simulink model "EChacks1"  (R2018a)
settings: Solver=FixedStepAuto  StartTime=0.0  StopTime=inf  RelTol=1e-3  EnableMultiTasking=on
PreLoadFcn:
  | Ts = 0.01;
  | Ts_wifi = 0.1;
libraries: arduinosensorlib x2, simulink x1
settings Model: SimulationMode=external  ExtModeTrigDuration=2  Creator=bnewman  LastModifiedBy=niuniusongqiang
settings OptimizationCC: PassReuseOutputArgsThreshold=0  MaxStackSize=64
settings DebuggingCC: ParameterTunabilityLossMsg=error
settings HardwareCC: ProdBitPerPointer=32  ProdBitPerSizeT=32  ProdBitPerPtrDiffT=32  ProdLargestAtomicInteger=Long  ProdLargestAtomicFloat=Double  ProdWordSize=32  ProdHWDeviceType=ARM Compatible->ARM Cortex  UseEmbeddedCoderFeatures=off  UseSimulinkCoderFeatures=off
settings SFSimCC: MATLABDynamicMemAlloc=off
settings RTWCC: SystemTargetFile=ert.tlc  HardwareBoard=Arduino MKR1000  TLCOptions=-aInlineSetEventsForThisBaseRateFcn=TLC_FALSE -aSuppressMultiTaskScheduler=TLC_FALSE -aRateBasedStepFcn=1  TemplateMakefile=ert_default_tmf  GenerateReport=on  Toolchain=Arduino ARM  BuildConfiguration=Faster Runs  LaunchReport=on
settings CodeAppCC: ForceParamTrailComments=on  OperatorAnnotations=on
settings ERTTargetCC: ERTCustomFileBanners=off  SupportContinuousTime=on  SupportNonInlinedSFcns=on  RemoveResetFunc=off  SupportVariableSizeSignals=on  ModelStepFunctionPrototypeControlCompliant=off

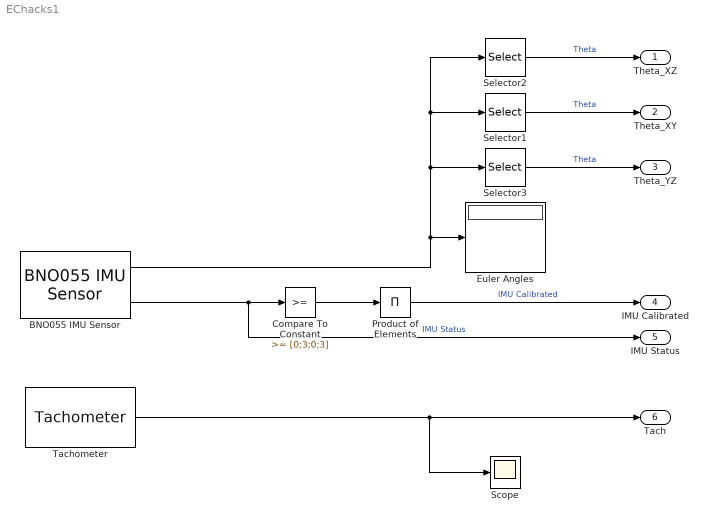
== system EChacks1 ==
  BNO055 IMU Sensor : arduinosensorlib/BNO055 IMU Sensor  SlaveAddress=0x28  OperationMode=Fusion  SlaveAddress_=hex2dec( '28' )  Accel=off  AngularRate=off  MagField=off  EulerAngles=on  Quat=off  LinearAccel=off  GravityVector=off  AccelRange=4G  AccelBW=62.5 Hz  GyroRange=2000 dps  GyroBW=32 Hz  MagODR=10 Hz  SampleTime=0.01
      settings: SourceProductName=Simulink Support for Arduino Sensors
  Compare To Constant : simulink/Logic and Bit Operations/Compare To Constant  relop=>=  const=[0;3;0;3]  OutDataTypeStr=boolean
  Euler Angles : Display
  Product of Elements : Product  Inputs=*
  Scope : Scope
  Selector1 : Selector  InputPortWidth=3  IndexOptions=Index vector (dialog)  Indices=2  OutputSizes=1
  Selector2 : Selector  InputPortWidth=3  IndexOptions=Index vector (dialog)  Indices=1  OutputSizes=1
  Selector3 : Selector  InputPortWidth=3  IndexOptions=Index vector (dialog)  Indices=3  OutputSizes=1
  Tachometer : arduinosensorlib/Tachometer  PinNumber=16  InterruptMode=RISING  SampleTime=0.1
      settings: SourceProductName=Simulink Support for Arduino Sensors
  Theta_XZ : Outport
  Theta_XY : Outport  Port=2
  Theta_YZ : Outport  Port=3
  IMU Calibrated : Outport  Port=4
  IMU Status : Outport  Port=5
  "Tach " : Outport  Port=6
  wires:
  BNO055 IMU Sensor/2 -> IMU Status/1, Compare To Constant/1  "IMU Status"
  BNO055 IMU Sensor/1 -> Euler Angles/1, Selector3/1, Selector2/1, Selector1/1
  Compare To Constant/1 -> Product of Elements/1
  Selector2/1 -> Theta_XZ/1  "Theta"
  Product of Elements/1 -> IMU Calibrated/1  "IMU Calibrated"
  Selector1/1 -> Theta_XY/1  "Theta"
  Selector3/1 -> Theta_YZ/1  "Theta"
  Tachometer/1 -> Scope/1, "Tach "/1
